simulink subsystem "UAV_2010_Model"  (R2023b)
settings: Solver=VariableStepAuto  StartTime=0.0  StopTime=10.0  RelTol=1e-3
settings Model: Creator=aarongreisen  LastModifiedBy=aarongreisen

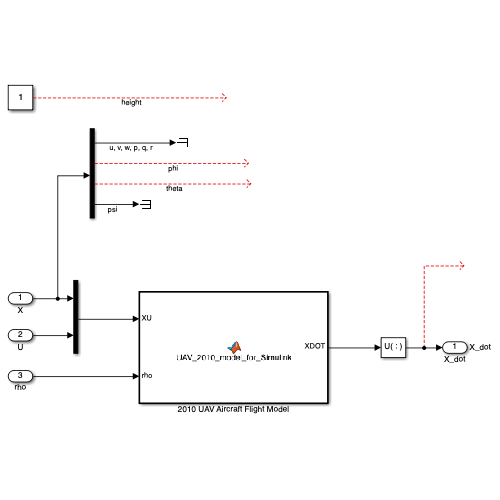
[thumbnail: Simulink's stored preview of the top-level diagram]
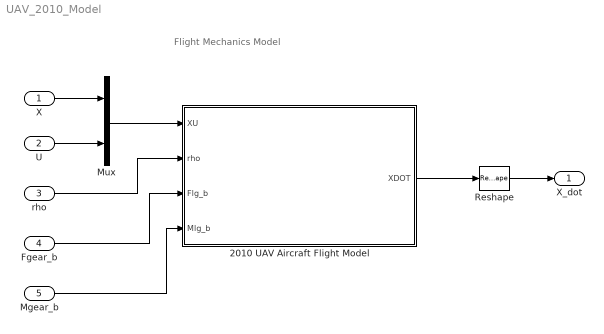
== system UAV_2010_Model ==
  note: Flight Mechanics Model
  X : Inport
  U : Inport  Port=2
  rho : Inport  Port=3
  Fgear_b : Inport  Port=4
  Mgear_b : Inport  Port=5
  2010 UAV Aircraft Flight Model : MATLAB Function  TreatAsAtomicUnit=on
  Mux : Mux  Inputs=[9 4]
  Reshape : Reshape
  X_dot : Outport  SignalName=X_dot
  wires:
  rho/1 -> 2010 UAV Aircraft Flight Model/2(rho)
  Reshape/1 -> X_dot/1
  Mux/1 -> 2010 UAV Aircraft Flight Model/1(XU)
  2010 UAV Aircraft Flight Model/1(XDOT) -> Reshape/1
  X/1 -> Mux/1
  U/1 -> Mux/2
  Fgear_b/1 -> 2010 UAV Aircraft Flight Model/3(Flg_b)
  Mgear_b/1 -> 2010 UAV Aircraft Flight Model/4(Mlg_b)

== matlab function UAV_2010_Model/2010 UAV Aircraft Flight Model ==
  data: XU input; XDOT output; rho input; Flg_b input; Mlg_b input
function XDOT  = UAV_2010_model_for_Simulink(XU, rho, Flg_b, Mlg_b)

%------------------STATE AND CONTROL VECTOR--------------------------------
% Extract state vector
x1 = XU(1); % u
x2 = XU(2); % v
x3 = XU(3); % w
x4 = XU(4); % p
x5 = XU(5); % q
x6 = XU(6); % r
x7 = XU(7); % phi
x8 = XU(8); % theta
x9 = XU(9); % psi

U = XU(10:13);

u1 = U(1); %d_A (aileron)
u2 = U(2); %d_T (stabilizer)
u3 = U(3); %d_R (rudder)
u4 = U(4); %d_th1 (throttle 1)

%---------------------CONSTANTS--------------------------------------------
% Nominal vehicle constants
m = 16.55612;            % Aircraft total mass (kg)

cbar = 0.7020814;        % Mean Aerodynamic Chord (m)
S = 1.309933;            % Wing planform area

Xcg = 0.2*cbar;          % x position of CoG in Fm (m)
Ycg = 0*cbar;            % y position of CoG in Fm (m)
Zcg = -0.10*cbar;        % z position of CoG in Fm (m)

% Engine constants
Xapt1 = -0.3556;         % x position of engine 1 force in Fm (m)
Yapt1 = 0;               % x position of engine 1 force in Fm (m)
Zapt1 = -0.0508;         % x position of engine 1 force in Fm (m)

% Other constants
g = 9.81;                % grav constant

%---------------------1. CONTROL LIMITS/SATURATION-------------------------


%---------------------2. INTERMEDIATE VARIABLES----------------------------
% Calculate airspeed
Va = sqrt(x1^2 + x2^2 + x3^2);

% Calculate alpha and beta
alpha = atan2(x3,x1)*180/pi;
beta = asin(x2/Va)*180/pi;

% Calculate dynamic pressure
Q = 0.5*rho*Va^2;

% Define vectors wbe_b and V_b
wbe_b = [x4;x5;x6];
V_b = [x1;x2;x3];

%---------------------3. AERODYNAMIC FORCE COEFFICIENTS--------------------
% Calculate the CL_wb

CL_noElev = -0.00002271*alpha^3 - 0.0002302*alpha^2 + 0.06565*alpha + 0.03959; % CL

CL_elevEffect = (-0.00001250958*alpha^3 + 0.000007639437*alpha^2 + 0.000286478898*alpha + 0.625574419317)*u2; % elevator effect on lift

% Total lift force coefficient
CL = CL_noElev + CL_elevEffect;  

% Total drag force
CD = 0.000857*alpha^2 - 0.0004961*alpha + 0.0217;   % Curve fit of CD vs alpha

% % Total side force
if beta > 30.857                                    % piecewise parametrization of side force coefficient
    CY = 0.004409*beta -0.1694;
elseif beta <= 30.857 && beta >= -30.857
    CY = -0.001126*beta + 0.001396;
else
    CY = 0.004409*beta -0.1694;
end
%---------------------4. DIMENSIONAL AERODYNAMIC FORCES--------------------
% Calculate the actual dimensional forces in F_s (stability axis)
FA_s = [-CD*Q*S;
        CY*Q*S;
        -CL*Q*S];

rad = pi/180;

C_bs = [cos(alpha*rad) 0 -sin(alpha*rad);
        0 1 0;
        sin(alpha*rad) 0 cos(alpha*rad)];

FA_b = C_bs*FA_s;

%---------------------5. AERODYNAMIC MOMENT COEFFICIENT ABOUT CG --------------------
% Calculate CM = [Cl;Cm;Cn] about aerodynamic center in Fb

if beta > -17.409 && beta < 17.409                       % piecewise parameterization of CR
    eta11 = -0.0001058*(beta) + 0.0002933;
elseif beta <= -17.409
    eta11 = 0.0005473*beta + 0.01108;
else 
    eta11 = 0.0005473*beta -0.01108;
end

eta21 = CMBA_lookup_table_2010_UAV(alpha, beta);           % CM lookup table
eta31 = CNBA_lookup_2010_UAV(beta);                        % CN lookup table

CMcg_b = [eta11 - 0.02864*u1 + dCRBA_dRudder(u3, alpha);       % all moments about CG in body axis including control surface effectiveness
          eta21 + dCMSA_dElevator(u2, alpha, beta);
          eta31 + dCNBA_dRudder(alpha, u3)];

%---------------------6. AERODYNAMIC MOMENT ABOUT CG --------------------
% Normalize to an aerodynamic moment
MAcg_b = CMcg_b*Q*S*cbar;

% %---------------------7. AERODYNAMIC  COEFFICIENT ABOUT CG --------------------------
% rcg_b = [Xcg;Ycg;Zcg];
% rac_b = [Xac;Yac;Zac];
% MAcg_b = MAac_b + cross(FA_b,rcg_b - rac_b);

%---------------------8. ENGINE FORCE AND MOMENT ------------------------------------
% effect of engine. First, calculate thrust of engine
% engine_coeffs = [1.012e-09, -5.527e-05, 1.044];
% 
% RPM = 158000*u4;
% if u4 > 1
%     RPM = 158000;
% end
% if RPM >= 0
%     F1 = (engine_coeffs(1)*RPM^2 + engine_coeffs(2)*RPM + engine_coeffs(3))*4.44822;
% else
%     F1 = 0;
% end

F1 = u4*m*g;

% assuming engine thrust is aligned with Fb, we have
FE1_b = [F1;0;0];
FE_b = FE1_b;

% engine moment due to offset of engine thrust from CoG
mew1 = [Xcg - Xapt1;
        Yapt1 - Ycg;
        Zcg - Zapt1];

MEcg1_b = cross(mew1,FE1_b);

MEcg_b = MEcg1_b;

%---------------------8.5. LANDING GEAR FORCE AND MOMENT ----------------------


%---------------------9. GRAVITY EFFECTS ------------------------------------
% Calculate gravitational forces in the body frame. This causes no moment
% about CoG
g_b = [-g*sin(x8);
        g*cos(x8)*sin(x7);
        g*cos(x8)*cos(x7)];

Fg_b = m*g_b;

%---------------------10. GRAVITY EFFECTS ------------------------------------
% Inertia matrix
Ib = [1.1619 0 -0.0607;
        0 5.6276 0;
        -0.0607 0 6.1040];

% Inverse of inertia matrix
% symmetric about xz plane
invIb =    [0.861106618696125	0	                0.00856310153257778
            0	                0.177695642902836	0
            0.00856310153257778	0	                0.163912152729854];

% Form R_b (all forces in Fb) and calculate udot, vdot, wdot
F_b = Fg_b + FE_b + FA_b + Flg_b;
x1to3dot = (1/m)*F_b - cross(wbe_b,V_b);

% Form Mcg_b (all moments about CoG in Fb) and calculate pdot, qdot, rdot
Mcg_b = MAcg_b + MEcg_b + Mlg_b;
x4to6dot = invIb*(Mcg_b - cross(wbe_b,Ib*wbe_b));

% Calculate phidot, thetadot, psidot
H_phi = [1 sin(x7)*tan(x8) cos(x7)*tan(x8);
         0 cos(x7) -sin(x7);
         0 sin(x7)/cos(x8) cos(x7)/cos(x8)];

x7to9dot = H_phi*wbe_b;

% Place in first order form
XDOT = [x1to3dot; 
        x4to6dot; 
        x7to9dot];

%     function tan = atan2_0_pi(y,x)
%         if x == 0
%             if y == 0
%                 tan = 0;
%             elseif y > 0
%                 tan = pi/2;
%             else
%                 tan = 3*pi/3;
%             end
%         elseif x > 0
%             if y >= 0
%                 tan = atan(y/x);
%             else
%                 tan = atan(y/x) + 2*pi;
%             end
%         elseif x < 0
%             if y == 0
%                 tan = pi;
%             else
%                 tan = atan(y/x) + pi;
%             end
%         end
%     end

end
